simulink model "tip_interaction"  (R2016b)
settings: Solver=VariableStepAuto  StartTime=0.0  StopTime=trun  RelTol=1e-9  AbsTol=1e-9
values from neighbouring files (symbols this model uses):
  Ki = 0.01    [force_sim2.m]
libraries: simulink x1
settings Model: Creator=arnold  LastModifiedBy=arnold

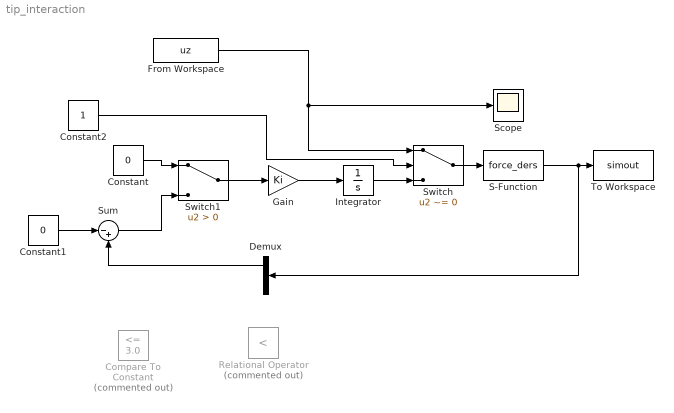
== system tip_interaction ==
  Compare To Constant : simulink/Logic and Bit Operations/Compare To Constant  Commented=on  relop=<=  const=3.0  OutDataTypeStr=boolean
  Constant : Constant  Value=0
  Constant1 : Constant  Value=0
  Constant2 : Constant
  Demux : Demux  Outputs=2
  From Workspace : FromWorkspace  VariableName=uz  SampleTime=0
  Gain : Gain  Gain=Ki
  Integrator : Integrator
  Relational Operator : RelationalOperator  Commented=on  Operator=<  OutDataTypeStr=boolean  RndMeth=Simplest
  S-Function : S-Function  FunctionName=force_ders  Parameters=params  SFunctionDeploymentMode=off  EnableBusSupport=off
  Scope : Scope
  Sum : Sum  Inputs=|-+
  Switch : Switch  Criteria=u2 ~= 0
  Switch1 : Switch  Criteria=u2 > Threshold
  To Workspace : ToWorkspace  VariableName=simout  SaveFormat=Timeseries  SampleTime=-1
  wires:
  S-Function/1 -> Demux/1, To Workspace/1
  From Workspace/1 -> Switch/1, Scope/1
  Gain/1 -> Integrator/1
  Switch/1 -> S-Function/1
  Integrator/1 -> Switch/3
  Switch1/1 -> Gain/1
  Constant/1 -> Switch1/1
  Sum/1 -> Switch1/3
  Constant1/1 -> Sum/1
  Demux/1 -> Sum/2
  Constant2/1 -> Switch/2
